simulink model "testBalancing"  (R2021a)
settings: Solver=FixedStepAuto  StartTime=0.0  StopTime=inf  FixedStep=0.01  RelTol=1e-3
undefined symbols (not defined in the file): SystemState_t
libraries: fl_lib x2, nesl_utility x2
settings Model: Creator=Carlo Edoardo  LastModifiedBy=Carlo Edoardo

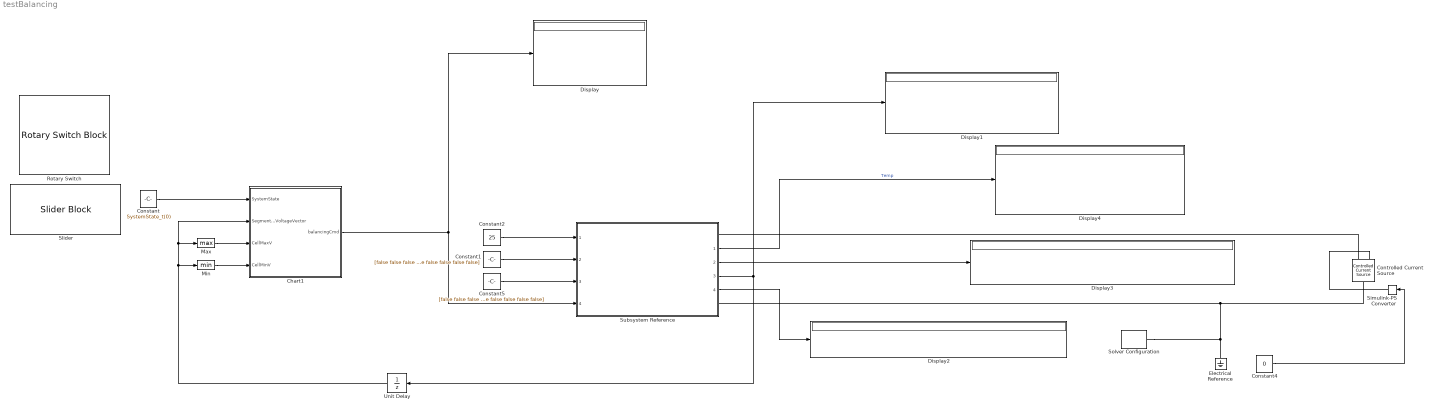
== system testBalancing ==
  Chart1 : Stateflow chart  TreatAsAtomicUnit=on
  Constant : Constant  Value=SystemState_t(0)  OutDataTypeStr=Enum: SystemState_t
  Constant1 : Constant  Value=[false false false false false false false false false false]
  Constant2 : Constant  Value=25  OutDataTypeStr=double
  Constant4 : Constant  Value=0
  Constant5 : Constant  Value=[false false false false false false false false false false]
  Controlled Current Source : fl_lib/Electrical/Electrical Sources/Controlled Current Source
  Display{,1..4} (5 alike) : Display
  Electrical Reference : fl_lib/Electrical/Electrical Elements/Electrical Reference
  Max : MinMax  Function=max
  Min : MinMax
  Rotary Switch : RotarySwitchBlock  UseEnumeratedDataType=on  EnumeratedDataType=SystemState_t
      settings: Values={{'Parking', 'Driving', 'Charging', 'Balancing'}, [0 1 2 3]}
  Simulink-PS Converter : nesl_utility/Simulink-PS Converter  PhysicalDomain=network_engine_domain  SubClassName=ps_input  LeftPortType=input  RightPortType=output  PseudoPeriodic=off  Frequencies=[]  NoiseDistribution=none  NoiseParameters=[]  Unit=1  AffineConversion=off  FilteringAndDerivatives=provide  SimscapeFilterOrder=1  InputFilterTimeConstant=0.001  UdotUserProvided=0
      settings: SourceProductBaseCode=PW,SS
  Slider : SliderBlock
  Solver Configuration : nesl_utility/Solver Configuration  PhysicalDomain=network_engine_domain  SubClassName=solver  LeftPortType=input  RightPortType=generic  Tones=[]  Harmonics=[]  SimulateNoise=off  Profile=off  UseLocalSampling=off  EnableSwitchedLinearOptims=on  FrequencyDomain=off  UseCCode=off  RelTol=0.001  AbsTol=1e-06  MinStep=1e-09  ToWorkspace=off  RevertToSquareIcSolve=off  NumHomotopyIterations=100  PhasorMode=off  PhasorModeNumHarmonics=1  DoDC=off  ResidualTolerance=1e-09  UseLocalSolver=off  LocalSolverChoice=NE_BACKWARD_EULER_ADVANCER  LocalSolverSampleTime=0.001  DoFixedCost=off  MaxNonlinIter=3  MaxModeIter=2  ComputeImpulses=off  ImpulseIterations=2  LinearAlgebra=auto  EquationFormulation=NE_TIME_EF  DelaysMemoryBudget=1024  AutomaticFiltering=on  FilteringTimeConstant=0.001  PartitionStorageMethod=AS_NEEDED  PartitionMemoryBudget=1024  PartitionMethod=ROBUST
      settings: SourceProductBaseCode=PW,SS
  Subsystem Reference : Subsystem  ReferencedSubsystem=battery_module
      settings: PortSchema="{\"entries\":[{\"content\":{\"sides\":[{\"content\":{\"connectorIds\":[\"In1\",\"In2\",\"In3\",\"In4\"]},\"type\":\"ConnectorPlacement.EquallySpacedRectSide\",\"uuid\":\"f42d6b3d-39c7-468b-a9a7-4e5d796eba3b\"},{\"content\":{\"connectorIds\":[\"RConn1\",\"Out1\",\"Out2\",\"Out3\",\"Out4\",\"RConn2\"],\"side\":\"RIGHT\"},\"type\":\"ConnectorPlacement.EquallySpacedRectSide\",\"uuid\":\"e762e236-7776-43b9-bd8d-fb7f2716d190\"},{\"content\":{\"connectorIds\":[],\"side\":\"TOP\"},\"type\":\"ConnectorPlacement.EquallySpacedRectSide\",\"uuid\":\"bd0c4b53-2dd2-497f-95b6-77c2ca394183\"}]},\"type\":\"ConnectorPlacement.EquallySpacedConnector\",\"uuid\":\"abacbee7-c859-4f21-9973-420371fecb92\"}],\"packageUris\":[\"http://schema.mathworks.com/mf0/Connector/R2020b\"],\"version\":\"1.0\"}"
  Unit Delay : UnitDelay  SampleTime=-1  HasFrameUpgradeWarning=on
  wires:
  Max/1 -> Chart1/3(CellMaxV)
  Min/1 -> Chart1/4(CellMinV)
  Constant/1 -> Chart1/1(SystemState)
  Unit Delay/1 -> Chart1/2(SegmentVoltageVector), Max/1, Min/1
  Chart1/1(balancingCmd) -> Subsystem Reference/4, Display/1
  Constant2/1 -> Subsystem Reference/1
  Subsystem Reference/3 -> Unit Delay/1, Display1/1
  Constant1/1 -> Subsystem Reference/2
  Subsystem Reference/4 -> Display2/1
  Subsystem Reference/2 -> Display3/1
  Constant4/1 -> Simulink-PS Converter/1
  Subsystem Reference/1 -> Display4/1  "Temp"
  Constant5/1 -> Subsystem Reference/3
  connections:
  Simulink-PS Converter/RConn1 -- Controlled Current Source/RConn1
  Solver Configuration/RConn1 -- Electrical Reference/LConn1 -- Controlled Current Source/LConn1 -- Subsystem Reference/RConn2
  Controlled Current Source/RConn2 -- Subsystem Reference/RConn1

== stateflow chart testBalancing/Chart1 ==
  state OFF
    en:
    balancingCmd(:)=0;
    en,du:
    DeltaVCell = CellMaxV - CellMinV;
  state ON
    state Balancing
      en, du:
      balancingCmd = ((SegmentVoltageVector - CellMinV) > DeltaVTargetMin);
      flagBalancingDone=all(~balancingCmd)
    state WaitRelaxation
      en: balancingCmd(:)=0;
    state BalancingFinished
      DeltaVCell=CellMaxV-CellMinV;
    state MeasureVoltage
      DeltaVCell=CellMaxV-CellMinV;
    (default) -> Balancing
    Balancing -> WaitRelaxation [order 2] : [(flagBalancingDone  ==  0)&&...
        | after(800,msec)]
    MeasureVoltage -> Balancing
    WaitRelaxation -> MeasureVoltage : after(1000, msec)
    Balancing -> BalancingFinished [order 1] : [flagBalancingDone  ==  1]
    BalancingFinished -> Balancing : [DeltaVCell > DeltaVTargetMin]
  (default) -> OFF
  ON -> OFF : [SystemState ~=  Balancing]
  OFF -> ON : [(SystemState==Balancing) && ...
      | DeltaVCell > DeltaVTargetMin]
  data: SystemState input Enum: SystemState_t; SegmentVoltageVector input size=10; DeltaVTargetMin parameter; balancingCmd output; CellMaxV input; CellMinV input; flagBalancingDone local; DeltaVCell local
